simulink model "soc_dvbs2_fpga"  (R2025b)
settings: Solver=FixedStepDiscrete  StartTime=0.0  StopTime=0  RelTol=1e-3
InitFcn:
  | soc_dvbs2_init;
values from neighbouring files (symbols this model uses):
  Rsym = 4e6    (= 4000000)    [soc_dvbs2_init.m]
  soc_dvbs2_txPacketBits = [1 1 0 1 0 1 1 1 0 1 1 1 ... (2972 elements, 2972x1)]    [soc_dvbs2_txPacketBits.mat]
  syncWord = (dec2bin(hex2dec('AC')) - '0').'    [soc_dvbs2_init.m]
  txDataOut = txobj(frameBits(:))    [soc_dvbs2_init.m]
  txFiltCoeff = txobj.pTxFilterCoeff    [soc_dvbs2_init.m]
undefined symbols (not defined in the file or in its folder): Add, coefficientsLog, coefficientsSqrt1, coefficientsSqrt2, dataBits, designMultirateFIR, noisePow, NumBits1, NumBits2, seedsURNG1, seedsURNG2, Shift, Slope1, Slope2, soc_dvbs2_designFIRFilter, txDataOutS1, txDataOutS10, txDataOutS12, txDataOutS13, txDataOutS14, txDataOutS15, txDataOutS16, txDataOutS18, txDataOutS19, txDataOutS2, txDataOutS20, txDataOutS21, txDataOutS22, txDataOutS24, txDataOutS25, txDataOutS26, txDataOutS27, txDataOutS3, txDataOutS4, txDataOutS5, txDataOutS6, txDataOutS7, txDataOutS8, txDataOutS9
libraries: simulink x214, hdlsllib x211, dspsigops x22, dsphdlfiltering2 x8, dsphdlsigops2 x5, commseqgen3 x5, dsphdlmathfun2 x3, hwlogicconnlib x2, whdledac x2, commhdlcrc x2, whdlutilities x1, whdlmod x1
(part 2 of 12)

== system soc_dvbs2_fpga/DVBS2/DVBS2 TxRx/DVB-S2 HDL Receiver/No HDL2 ==
  UPL : Inport
  DFL : Inport  Port=2
  SYNC : Inport  Port=3
  SYNCD : Inport  Port=4
  frameStart : Inport  Port=5
  frameEnd : Inport  Port=6
  To Workspace : ToWorkspace  VariableName=simUPL  SampleTime=-1
      settings: Save2DSignal=2-D array (concatenate along first dimension)
  To Workspace1 : ToWorkspace  VariableName=simDFL  SampleTime=-1
      settings: Save2DSignal=2-D array (concatenate along first dimension)
  To Workspace2 : ToWorkspace  VariableName=simSYNC  SampleTime=-1
      settings: Save2DSignal=2-D array (concatenate along first dimension)
  To Workspace3 : ToWorkspace  VariableName=simSYNCD  SampleTime=-1
      settings: Save2DSignal=2-D array (concatenate along first dimension)
  To Workspace4 : ToWorkspace  VariableName=simFrameStart  SampleTime=-1
      settings: Save2DSignal=2-D array (concatenate along first dimension)
  To Workspace5 : ToWorkspace  VariableName=simFrameEnd  SampleTime=-1
      settings: Save2DSignal=2-D array (concatenate along first dimension)
  wires:
  DFL/1 -> To Workspace1/1
  SYNCD/1 -> To Workspace3/1
  UPL/1 -> To Workspace/1
  SYNC/1 -> To Workspace2/1
  frameStart/1 -> To Workspace4/1
  frameEnd/1 -> To Workspace5/1

== system soc_dvbs2_fpga/DVBS2/DVBS2 TxRx/DVB-S2 HDL Receiver/Stream Recovery ==
  bitsIn : Inport  OutDataTypeStr=boolean  PortDimensions=[1 1]  SampleTime=1/(Rsym*32)
  startIn : Inport  Port=2  OutDataTypeStr=boolean  PortDimensions=[1 1]
  validIn : Inport  Port=3  OutDataTypeStr=boolean  PortDimensions=[1 1]
  BB Decoder : Subsystem
      settings: PortSchema="{\"entries\":[{\"content\":{\"sides\":[{\"content\":{\"connectorIds\":[\"In1\",\"In2\",\"In3\",\"In4\",\"In5\",\"In6\",\"In7\",\"In8\"]},\"type\":\"ConnectorPlacement.EquallySpacedRectSide\",\"uuid\":\"2ee8952a-ba35-4074-ae69-b380b0fca75a\"},{\"content\":{\"connectorIds\":[\"Out1\",\"Out2\",\"Out3\",\"Out4\",\"Out5\",\"Out6\",\"Out7\",\"Out8\",\"Out9\",\"Out10\",\"Out11\",\"Out12\",\"Out13\",\"Out14\",\"Out15\",\"Out16\",\"Out17\"],\"side\":\"RIGHT\"},\"type\":\"ConnectorPlacement.EquallySpacedRectSide\",\"uuid\":\"5cd54040-f4d2-41eb-8bc9-10e507694db5\"},{\"content\":{\"connectorIds\":[\"Out18\",\"Out19\",\"Out20\"],\"side\":\"TOP\"},\"type\":\"ConnectorPlacement.EquallySpacedRectSide\",\"uuid\":\"7ef39af9-18b6-4154-ba4c-25b08baa09fa\"}]},\"type\":\"ConnectorPlacement.EquallySpacedConnector\",\"uuid\":\"52807250-24d4-4e44-a1d7-a664e63f1684\"}],\"packageUris\":[\"http://schema.mathworks.com/mf0/Connector/R2020b\"],\"version\":\"1.0\"}"
  BB Demultiplexer : Subsystem
  BB Descrambler : Subsystem
  BB Header CRC Check : Subsystem
  Delay{1..2,4..9,11..15,17..18,20..24} (20 alike) : Delay  DelayLength=1
  bitsOut : Outport  OutDataTypeStr=boolean  PortDimensions=[1 1]
  startOut : Outport  Port=2  OutDataTypeStr=boolean  PortDimensions=[1 1]
  endOut : Outport  Port=3  OutDataTypeStr=boolean  PortDimensions=[1 1]
  validOut : Outport  Port=4  OutDataTypeStr=boolean  PortDimensions=[1 1]
  errorOut : Outport  Port=5  OutDataTypeStr=boolean  PortDimensions=[1 1]
  invalidPkt : Outport  Port=6  OutDataTypeStr=boolean  PortDimensions=[1 1]
  headerCRCInfo : Outport  Port=7  OutDataTypeStr=fixdt(0,2,0)  PortDimensions=[1 1]
  TSorGS : Outport  Port=8  OutDataTypeStr=fixdt(0,2,0)  PortDimensions=[1 1]
  SISorMIS : Outport  Port=9  OutDataTypeStr=boolean  PortDimensions=[1 1]
  CCMorACM : Outport  Port=10  OutDataTypeStr=boolean  PortDimensions=[1 1]
  ISSYI : Outport  Port=11  OutDataTypeStr=boolean  PortDimensions=[1 1]
  NPD : Outport  Port=12  OutDataTypeStr=boolean  PortDimensions=[1 1]
  RO : Outport  Port=13  OutDataTypeStr=fixdt(0,2,0)  PortDimensions=[1 1]
  MIS_ISI : Outport  Port=14  OutDataTypeStr=uint8  PortDimensions=1
  UPL : Outport  Port=15  OutDataTypeStr=uint16  PortDimensions=1
  DFL : Outport  Port=16  OutDataTypeStr=uint16  PortDimensions=1
  SYNC : Outport  Port=17  OutDataTypeStr=uint8  PortDimensions=1
  SYNCD : Outport  Port=18  OutDataTypeStr=uint16  PortDimensions=1
  frameSrt : Outport  Port=19  OutDataTypeStr=boolean  PortDimensions=[1 1]
  frameEnd : Outport  Port=20  OutDataTypeStr=boolean  PortDimensions=[1 1]
  wires:
  bitsIn/1 -> Delay1/1
  BB Demultiplexer/2(dValidOut) -> Delay20/1
  BB Demultiplexer/6(hvalidOut) -> Delay24/1
  BB Decoder/5(errorOut) -> errorOut/1
  BB Decoder/4(validOut) -> validOut/1
  BB Decoder/1(bitsOut) -> bitsOut/1
  Delay9/1 -> BB Decoder/1(dstartIn)
  BB Descrambler/1(bitsOut) -> Delay7/1
  Delay14/1 -> BB Decoder/8(herrorIn)
  BB Decoder/8(SISorMIS) -> SISorMIS/1
  BB Header CRC Check/3(dbitsOut) -> Delay8/1
  Delay11/1 -> BB Decoder/2(dvalidIn)
  Delay8/1 -> BB Decoder/3(dbitsIn)
  BB Decoder/15(DFL) -> DFL/1
  BB Header CRC Check/8(herrorOut) -> Delay14/1
  Delay12/1 -> BB Decoder/7(validIn)
  BB Decoder/17(SYNCD) -> SYNCD/1
  BB Header CRC Check/4(hbitsOut) -> Delay13/1
  BB Decoder/11(NPD) -> NPD/1
  BB Demultiplexer/4(hstartOut) -> Delay22/1
  BB Decoder/12(RO) -> RO/1
  BB Demultiplexer/5(hendOut) -> Delay23/1
  BB Demultiplexer/1(dstartOut) -> Delay18/1
  BB Descrambler/3(validOut) -> Delay17/1
  validIn/1 -> Delay6/1
  BB Header CRC Check/7(hvalidOut) -> Delay12/1
  BB Decoder/14(UPL) -> UPL/1
  BB Decoder/3(endOut) -> endOut/1
  BB Decoder/9(CCMorACM) -> CCMorACM/1
  Delay4/1 -> BB Decoder/5(hstartIn)
  BB Demultiplexer/3(bitsOut) -> Delay21/1
  BB Descrambler/2(startOut) -> Delay15/1
  BB Header CRC Check/5(hstartOut) -> Delay4/1
  BB Header CRC Check/1(dstartOut) -> Delay9/1
  BB Decoder/2(startOut) -> startOut/1
  BB Decoder/10(ISSYI) -> ISSYI/1
  BB Header CRC Check/2(dvalidIn) -> Delay11/1
  BB Header CRC Check/6(hendOut) -> Delay5/1
  Delay5/1 -> BB Decoder/6(hendIn)
  Delay13/1 -> BB Decoder/4(hbitsIn)
  BB Decoder/13(MIS_ISI) -> MIS_ISI/1
  BB Decoder/16(SYNC) -> SYNC/1
  BB Decoder/7(TSorGS) -> TSorGS/1
  startIn/1 -> Delay2/1
  BB Decoder/18(invalidPkt) -> invalidPkt/1
  BB Decoder/6(headerCRCInfo) -> headerCRCInfo/1
  Delay1/1 -> BB Descrambler/1(bitsIn)
  Delay2/1 -> BB Descrambler/2(startIn)
  Delay6/1 -> BB Descrambler/3(validIn)
  Delay7/1 -> BB Demultiplexer/1(bitsIn)
  Delay15/1 -> BB Demultiplexer/2(startIn)
  Delay17/1 -> BB Demultiplexer/3(validIn)
  Delay18/1 -> BB Header CRC Check/1(dstartIn)
  Delay20/1 -> BB Header CRC Check/2(dValidIn)
  Delay21/1 -> BB Header CRC Check/3(bitsIn)
  Delay22/1 -> BB Header CRC Check/4(hstartIn)
  Delay23/1 -> BB Header CRC Check/5(hendIn)
  Delay24/1 -> BB Header CRC Check/6(hvalidIn)
  BB Decoder/19(frameStart) -> frameSrt/1
  BB Decoder/20(frameEnd) -> frameEnd/1

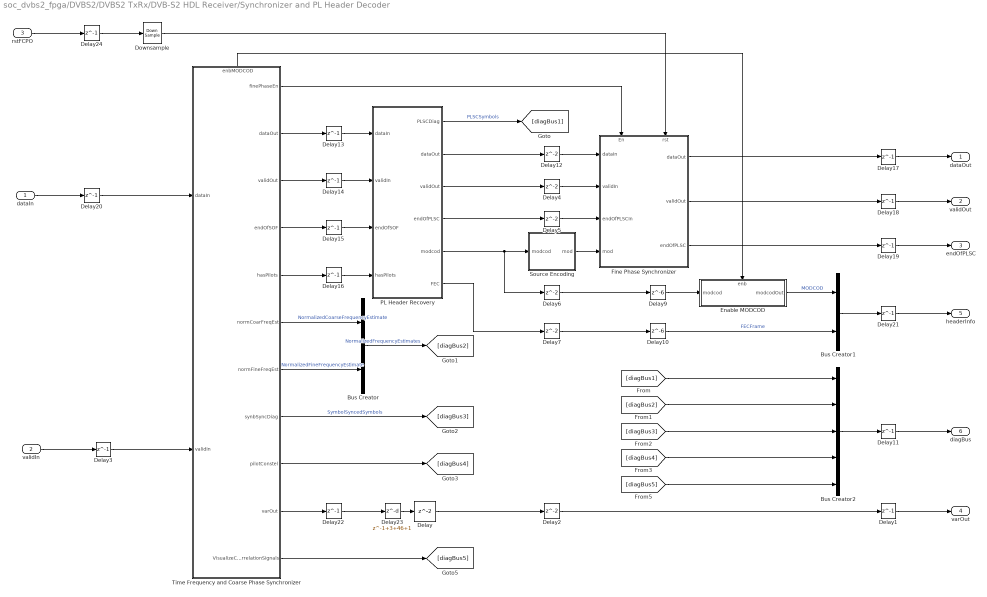
== system soc_dvbs2_fpga/DVBS2/DVBS2 TxRx/DVB-S2 HDL Receiver/Synchronizer and PL Header Decoder ==
  dataIn : Inport  OutDataTypeStr=fixdt(1,18,15)  PortDimensions=1  SampleTime=1/(Rsym*config.SamplesPerSymbol)
      settings: SignalType=complex
  validIn : Inport  Port=2  OutDataTypeStr=boolean  PortDimensions=1  SampleTime=1/(Rsym*config.SamplesPerSymbol)
  rstFCPO : Inport  Port=3  OutDataTypeStr=boolean  PortDimensions=1  SampleTime=1/(Rsym*config.SamplesPerSymbol)
  Bus Creator : BusCreator  Inputs=2
  Bus Creator1 : BusCreator  Inputs=2
  Bus Creator2 : BusCreator  Inputs=5
  Delay{,2,4..7,12} (7 alike) : Delay
  Delay{1,3,11,13..22,24} (14 alike) : Delay  DelayLength=1
  Delay10 : Delay  DelayLength=6
  Delay23 : Delay  DelayLength=1+3+46+1
  Delay9 : Delay  DelayLength=6
  Downsample : DownSample  N=config.SamplesPerSymbol  RateOptions=Allow multirate processing
  "Enable MODCOD " : Subsystem
      settings: PortSchema="{\"entries\":[{\"content\":{\"sides\":[{\"content\":{\"connectorIds\":[\"In1\"]},\"type\":\"ConnectorPlacement.EquallySpacedRectSide\",\"uuid\":\"e9d17376-cdb6-46fb-903f-9d282ad3c090\"},{\"content\":{\"connectorIds\":[\"Out1\"],\"side\":\"RIGHT\"},\"type\":\"ConnectorPlacement.EquallySpacedRectSide\",\"uuid\":\"a9734af5-b25e-45ab-96a0-7f27ff03e87c\"},{\"content\":{\"connectorIds\":[\"In2\"],\"side\":\"TOP\"},\"type\":\"ConnectorPlacement.EquallySpacedRectSide\",\"uuid\":\"cd34d4a9-2b51-417d-abe3-d9c0cedbfd72\"}]},\"type\":\"ConnectorPlacement.EquallySpacedConnector\",\"uuid\":\"3d42caf6-d237-4a2e-ba65-28be4744776a\"}],\"packageUris\":[\"http://schema.mathworks.com/mf0/Connector/R2020b\"],\"version\":\"1.0\"}"
      settings: LibrarySourceBlock=|
      | hdlsllib/Ports &
      | Subsystems/Subsystem
  Fine Phase Synchronizer : Subsystem
      settings: PortSchema="{\"entries\":[{\"content\":{\"sides\":[{\"content\":{\"connectorIds\":[\"In1\",\"In2\",\"In3\",\"In4\"]},\"type\":\"ConnectorPlacement.EquallySpacedRectSide\",\"uuid\":\"8cb05f70-3f7c-4fa6-8c33-963515007e67\"},{\"content\":{\"connectorIds\":[\"Out1\",\"Out2\",\"Out3\"],\"side\":\"RIGHT\"},\"type\":\"ConnectorPlacement.EquallySpacedRectSide\",\"uuid\":\"1928a8bf-9583-43f2-af59-80ea1a918df6\"},{\"content\":{\"connectorIds\":[\"In5\",\"In6\"],\"side\":\"TOP\"},\"type\":\"ConnectorPlacement.EquallySpacedRectSide\",\"uuid\":\"66048bc0-484a-4616-b173-7a52a6834176\"}]},\"type\":\"ConnectorPlacement.EquallySpacedConnector\",\"uuid\":\"51bb5bc9-87eb-4b94-8278-b6601d5ad231\"}],\"packageUris\":[\"http://schema.mathworks.com/mf0/Connector/R2020b\"],\"version\":\"1.0\"}"
  PL Header Recovery : Subsystem
  Source Encoding : Subsystem
  Time Frequency and Coarse Phase Synchronizer : Subsystem
      settings: PortSchema="{\"entries\":[{\"content\":{\"sides\":[{\"content\":{\"connectorIds\":[\"In1\",\"In2\"]},\"type\":\"ConnectorPlacement.EquallySpacedRectSide\",\"uuid\":\"4d277405-2c1f-464d-b6dc-b1e9ab229e6e\"},{\"content\":{\"connectorIds\":[\"Out1\",\"Out2\",\"Out3\",\"Out4\",\"Out5\",\"Out6\",\"Out7\",\"Out8\",\"Out9\",\"Out10\",\"Out11\"],\"side\":\"RIGHT\"},\"type\":\"ConnectorPlacement.EquallySpacedRectSide\",\"uuid\":\"271739cd-2ba1-4a70-9167-bfb95088c1ca\"},{\"content\":{\"connectorIds\":[\"Out12\"],\"side\":\"TOP\"},\"type\":\"ConnectorPlacement.EquallySpacedRectSide\",\"uuid\":\"6ccba931-85ed-495e-b91c-84f6ac00e636\"}]},\"type\":\"ConnectorPlacement.EquallySpacedConnector\",\"uuid\":\"210794f0-4960-4096-827d-5c263124cba0\"}],\"packageUris\":[\"http://schema.mathworks.com/mf0/Connector/R2020b\"],\"version\":\"1.0\"}"
  dataOut : Outport
  validOut : Outport  Port=2
  endOfPLSC : Outport  Port=3
  varOut : Outport  Port=4
  headerInfo : Outport  Port=5
  diagBus : Outport  Port=6
  wires:
  Bus Creator2/1 -> Delay11/1
  [diagBus4] -> Bus Creator2/4
  PL Header Recovery/6(FEC) -> Delay7/1
  Time Frequency and Coarse Phase Synchronizer/5(hasPilots) -> Delay16/1
  Time Frequency and Coarse Phase Synchronizer/10(varOut) -> Delay22/1
  Bus Creator1/1 -> Delay21/1
  Delay9/1 -> "Enable MODCOD "/1(modcod)
  rstFCPO/1 -> Delay24/1
  PL Header Recovery/5(modcod) -> Source Encoding/1(modcod), Delay6/1
  Delay13/1 -> PL Header Recovery/1(dataIn)
  [diagBus1] -> Bus Creator2/1
  Delay22/1 -> Delay23/1
  Delay19/1 -> endOfPLSC/1
  PL Header Recovery/3(validOut) -> Delay4/1
  [diagBus5] -> Bus Creator2/5
  Delay12/1 -> Fine Phase Synchronizer/1(dataIn)
  Delay10/1 -> Bus Creator1/2  "FECFrame"
  Fine Phase Synchronizer/1(dataOut) -> Delay17/1
  validIn/1 -> Delay3/1
  Fine Phase Synchronizer/3(endOfPLSC) -> Delay19/1
  PL Header Recovery/2(dataOut) -> Delay12/1
  Time Frequency and Coarse Phase Synchronizer/2(dataOut) -> Delay13/1
  dataIn/1 -> Delay20/1
  Time Frequency and Coarse Phase Synchronizer/11(VisualizeCorrelationSignals) -> [diagBus5]
  Delay7/1 -> Delay10/1
  Delay14/1 -> PL Header Recovery/2(validIn)
  Time Frequency and Coarse Phase Synchronizer/4(endOfSOF) -> Delay15/1
  Fine Phase Synchronizer/2(validOut) -> Delay18/1
  Delay5/1 -> Fine Phase Synchronizer/3(endOfPLSCIn)
  Delay3/1 -> Time Frequency and Coarse Phase Synchronizer/2(validIn)
  Delay/1 -> Delay2/1
  Time Frequency and Coarse Phase Synchronizer/3(validOut) -> Delay14/1
  Delay16/1 -> PL Header Recovery/4(hasPilots)
  [diagBus2] -> Bus Creator2/2
  Delay2/1 -> Delay1/1
  Delay15/1 -> PL Header Recovery/3(endOfSOF)
  Delay6/1 -> Delay9/1
  Delay17/1 -> dataOut/1
  PL Header Recovery/4(endOfPLSC) -> Delay5/1
  [diagBus3] -> Bus Creator2/3
  Delay4/1 -> Fine Phase Synchronizer/2(validIn)
  Source Encoding/1(mod) -> Fine Phase Synchronizer/4(mod)
  Delay18/1 -> validOut/1
  Time Frequency and Coarse Phase Synchronizer/8(synbSyncDiag) -> [diagBus3]  "SymbolSyncedSymbols"
  PL Header Recovery/1(PLSCDiag) -> [diagBus1]  "PLSCSymbols"
  Time Frequency and Coarse Phase Synchronizer/1(finePhaseEn) -> Fine Phase Synchronizer/5(En)
  Time Frequency and Coarse Phase Synchronizer/9(pilotConstel) -> [diagBus4]
  Delay1/1 -> varOut/1
  Delay20/1 -> Time Frequency and Coarse Phase Synchronizer/1(dataIn)
  Delay23/1 -> Delay/1
  Delay24/1 -> Downsample/1
  Delay11/1 -> diagBus/1
  Delay21/1 -> headerInfo/1
  Downsample/1 -> Fine Phase Synchronizer/6(rst)
  "Enable MODCOD "/1(modcodOut) -> Bus Creator1/1  "MODCOD"
  Time Frequency and Coarse Phase Synchronizer/12(enbMODCOD) -> "Enable MODCOD "/2(enb)
  Bus Creator/1 -> [diagBus2]  "NormalizedFrequencyEstimates"
  Time Frequency and Coarse Phase Synchronizer/6(normCoarFreqEst) -> Bus Creator/1  "NormalizedCoarseFrequencyEstimate"
  Time Frequency and Coarse Phase Synchronizer/7(normFineFreqEst) -> Bus Creator/2  "NormalizedFineFrequencyEstimate"

== system soc_dvbs2_fpga/DVBS2/DVBS2 TxRx/Digital Automatic Gain Control/Error Detector ==
  dataIn : Inport
  Add1 : Sum  Inputs=+-
  Complex to Real-Imag : ComplexToRealImag  Output=Real
  Conj : Math  Operator=conj
  Data Type Duplicate : DataTypeDuplicate
  Delay{,1,3..4} (4 alike) : Delay
  Product : Product
  Reference : Constant  Value=desiredOutputPower  OutDataTypeStr=Inherit: Inherit via back propagation  SampleTime=-1
  err : Outport
  wires:
  Complex to Real-Imag/1 -> Add1/2
  Product/1 -> Delay4/1
  Delay4/1 -> Complex to Real-Imag/1
  Delay3/1 -> err/1
  Delay1/1 -> Product/1
  Delay/1 -> Product/2
  Reference/1 -> Add1/1, Data Type Duplicate/1
  Conj/1 -> Delay/1
  dataIn/1 -> Conj/1, Data Type Duplicate/2, Delay1/1
  Add1/1 -> Delay3/1

== system soc_dvbs2_fpga/DVBS2/DVBS2 TxRx/Digital Automatic Gain Control/Loop Filter ==
  note: Fixed point precision loss warnings
      | are supressed in Mask Init Callback
  err : Inport
  Add : Sum  Inputs=|++  OutDataTypeStr=Inherit: Same as first input
  Delay1 : Delay  DelayLength=1
  Delay2 : Delay
  Delay3 : Delay
  Gain1 : Gain  Gain=stepSize  OutDataTypeStr=Inherit: Same as input
      mask init:
      | Simulink.suppressDiagnostic(gcb, 'SimulinkFixedPoint:util:fxpParameterPrecisionLoss');
  gain : Outport
  wires:
  Delay3/1 -> Gain1/1
  Delay2/1 -> Add/1
  Gain1/1 -> Delay2/1
  Add/1 -> Delay1/1
  Delay1/1 -> Add/2, gain/1
  err/1 -> Delay3/1

== system soc_dvbs2_fpga/DVBS2/DVBS2 TxRx/LUT Based Tx/Subsystem1 ==
  modcodidx : Inport
  enb : Inport  Port=2
  Delay : Delay  DelayLength=1
  From : From
  Goto : Goto
  HDL Counter : hdlsllib/Sources/HDL Counter  CountType=Count limited  CountInit=0  CountStep=1  CountMax=8370-1  CountFromType=Initial value  CountFrom=0  CountResetPort=off  CountLoadPort=off  CountEnbPort=on  CountDirPort=off  CountHitOutputPort=off  CountDataType=Unsigned  CountWordLen=32  CountFracLen=0  CountSampTime=1
  Logical Operator : Logic  Operator=OR  Inputs=4  AllPortsSameDT=off  OutDataTypeStr=boolean
  Multiport Switch : MultiPortSwitch  DataPortOrder=Zero-based contiguous  Inputs=24  DataPortForDefault=Additional data port  DiagnosticForDefault=Warning  zeroidx=on  SaturateOnIntegerOverflow=off  InputSameDT=off
  Subsystem : Subsystem
      settings: PortSchema="{\"entries\":[{\"content\":{\"sides\":[{\"content\":{\"connectorIds\":[\"In1\",\"In2\",\"In3\"]},\"type\":\"ConnectorPlacement.EquallySpacedRectSide\",\"uuid\":\"6ed0080d-8044-45ae-9509-1be5017662ca\"},{\"content\":{\"connectorIds\":[\"Out1\",\"Out2\",\"Out3\",\"Out4\",\"Out5\",\"Out6\"],\"side\":\"RIGHT\"},\"type\":\"ConnectorPlacement.EquallySpacedRectSide\",\"uuid\":\"674d766f-0d57-4001-a79f-bea5e47ca454\"},{\"content\":{\"connectorIds\":[\"Out7\"],\"side\":\"TOP\"},\"type\":\"ConnectorPlacement.EquallySpacedRectSide\",\"uuid\":\"4af606e0-b38a-47a9-8ca6-549744415caf\"}]},\"type\":\"ConnectorPlacement.EquallySpacedConnector\",\"uuid\":\"5c295423-4673-440c-afff-1364a30dca72\"}],\"packageUris\":[\"http://schema.mathworks.com/mf0/Connector/R2020b\"],\"version\":\"1.0\"}"
  Subsystem1 : Subsystem
      settings: PortSchema="{\"entries\":[{\"content\":{\"sides\":[{\"content\":{\"connectorIds\":[\"In1\",\"In2\",\"In3\"]},\"type\":\"ConnectorPlacement.EquallySpacedRectSide\",\"uuid\":\"6ed0080d-8044-45ae-9509-1be5017662ca\"},{\"content\":{\"connectorIds\":[\"Out1\",\"Out2\",\"Out3\",\"Out4\",\"Out5\",\"Out6\"],\"side\":\"RIGHT\"},\"type\":\"ConnectorPlacement.EquallySpacedRectSide\",\"uuid\":\"674d766f-0d57-4001-a79f-bea5e47ca454\"},{\"content\":{\"connectorIds\":[\"Out7\"],\"side\":\"TOP\"},\"type\":\"ConnectorPlacement.EquallySpacedRectSide\",\"uuid\":\"4af606e0-b38a-47a9-8ca6-549744415caf\"}]},\"type\":\"ConnectorPlacement.EquallySpacedConnector\",\"uuid\":\"5c295423-4673-440c-afff-1364a30dca72\"}],\"packageUris\":[\"http://schema.mathworks.com/mf0/Connector/R2020b\"],\"version\":\"1.0\"}"
  Subsystem2 : Subsystem
      settings: PortSchema="{\"entries\":[{\"content\":{\"sides\":[{\"content\":{\"connectorIds\":[\"In1\",\"In2\",\"In3\"]},\"type\":\"ConnectorPlacement.EquallySpacedRectSide\",\"uuid\":\"6ed0080d-8044-45ae-9509-1be5017662ca\"},{\"content\":{\"connectorIds\":[\"Out1\",\"Out2\",\"Out3\",\"Out4\",\"Out5\",\"Out6\"],\"side\":\"RIGHT\"},\"type\":\"ConnectorPlacement.EquallySpacedRectSide\",\"uuid\":\"674d766f-0d57-4001-a79f-bea5e47ca454\"},{\"content\":{\"connectorIds\":[\"Out7\"],\"side\":\"TOP\"},\"type\":\"ConnectorPlacement.EquallySpacedRectSide\",\"uuid\":\"4af606e0-b38a-47a9-8ca6-549744415caf\"}]},\"type\":\"ConnectorPlacement.EquallySpacedConnector\",\"uuid\":\"5c295423-4673-440c-afff-1364a30dca72\"}],\"packageUris\":[\"http://schema.mathworks.com/mf0/Connector/R2020b\"],\"version\":\"1.0\"}"
  Subsystem4 : Subsystem
      settings: PortSchema="{\"entries\":[{\"content\":{\"sides\":[{\"content\":{\"connectorIds\":[\"In1\",\"In2\",\"In3\"]},\"type\":\"ConnectorPlacement.EquallySpacedRectSide\",\"uuid\":\"6ed0080d-8044-45ae-9509-1be5017662ca\"},{\"content\":{\"connectorIds\":[\"Out1\",\"Out2\",\"Out3\",\"Out4\",\"Out5\",\"Out6\"],\"side\":\"RIGHT\"},\"type\":\"ConnectorPlacement.EquallySpacedRectSide\",\"uuid\":\"674d766f-0d57-4001-a79f-bea5e47ca454\"},{\"content\":{\"connectorIds\":[\"Out7\"],\"side\":\"TOP\"},\"type\":\"ConnectorPlacement.EquallySpacedRectSide\",\"uuid\":\"4af606e0-b38a-47a9-8ca6-549744415caf\"}]},\"type\":\"ConnectorPlacement.EquallySpacedConnector\",\"uuid\":\"5c295423-4673-440c-afff-1364a30dca72\"}],\"packageUris\":[\"http://schema.mathworks.com/mf0/Connector/R2020b\"],\"version\":\"1.0\"}"
  Terminator : Terminator
  Unit Delay Enabled Synchronous : hdlsllib/Discrete/Unit Delay Enabled Synchronous  InitialCondition=0.0  SampleTime=-1
  Out1 : Outport
  wires:
  Unit Delay Enabled Synchronous/1 -> Goto/1, Multiport Switch/1
  Multiport Switch/1 -> Out1/1
  modcodidx/1 -> Unit Delay Enabled Synchronous/1
  Delay/1 -> Subsystem2/1(rst), Subsystem4/1(rst), Subsystem1/1(rst), Subsystem/1(rst)
  enb/1 -> HDL Counter/1, Subsystem/2(enb), Subsystem2/2(enb), Subsystem4/2(enb), Subsystem1/2(enb)
  Subsystem/1(Out2) -> Multiport Switch/2, Multiport Switch/26
  Subsystem/2(Out3) -> Multiport Switch/3
  Subsystem/3(Out4) -> Multiport Switch/4
  Subsystem/4(Out5) -> Multiport Switch/5
  Subsystem/5(Out6) -> Multiport Switch/6
  Subsystem/6(Out7) -> Multiport Switch/7
  Subsystem1/1(Out2) -> Multiport Switch/8
  Subsystem1/2(Out3) -> Multiport Switch/9
  Subsystem1/3(Out4) -> Multiport Switch/10
  Subsystem1/4(Out5) -> Multiport Switch/11
  Subsystem1/5(Out6) -> Multiport Switch/12
  Subsystem1/6(Out7) -> Multiport Switch/13
  Subsystem4/1(Out2) -> Multiport Switch/14
  Subsystem4/2(Out3) -> Multiport Switch/15
  Subsystem4/3(Out4) -> Multiport Switch/16
  Subsystem4/4(Out5) -> Multiport Switch/17
  Subsystem4/5(Out6) -> Multiport Switch/18
  Subsystem4/6(Out7) -> Multiport Switch/19
  Subsystem2/1(Out2) -> Multiport Switch/20
  Subsystem2/2(Out3) -> Multiport Switch/21
  Subsystem2/3(Out4) -> Multiport Switch/22
  Subsystem2/4(Out5) -> Multiport Switch/23
  Subsystem2/5(Out6) -> Multiport Switch/24
  Subsystem2/6(Out7) -> Multiport Switch/25
  Logical Operator/1 -> Unit Delay Enabled Synchronous/2, Delay/1
  Subsystem/7(Out1) -> Logical Operator/1
  Subsystem4/7(Out1) -> Logical Operator/2
  Subsystem1/7(Out1) -> Logical Operator/3
  Subsystem2/7(Out1) -> Logical Operator/4
  From/1 -> Subsystem2/3(modcodidx), Subsystem4/3(modcodidx), Subsystem1/3(modcodidx), Subsystem/3(modcodidx)
  HDL Counter/1 -> Terminator/1

== system soc_dvbs2_fpga/DVBS2/DVBS2 TxRx/Channel/AWGN Generator/Gaussian Noise With Given Variance ==
  noiseVar : Inport
  x0 : Inport  Port=2
  x1 : Inport  Port=3
  Add1 : Sum  OutDataTypeStr=fixdt(1,16,11)
  Delay{1..9} (9 alike) : Delay
  Gain : Gain  Gain=1i
  Product1 : Product
  awgn : Outport
  wires:
  Add1/1 -> Delay3/1
  Product1/1 -> Delay1/1
  x1/1 -> Delay9/1
  x0/1 -> Delay8/1
  Gain/1 -> Delay5/1
  noiseVar/1 -> Delay7/1
  Delay1/1 -> awgn/1
  Delay2/1 -> Product1/1
  Delay3/1 -> Product1/2
  Delay4/1 -> Add1/1
  Delay5/1 -> Add1/2
  Delay6/1 -> Delay2/1
  Delay7/1 -> Delay6/1
  Delay8/1 -> Delay4/1
  Delay9/1 -> Gain/1

== system soc_dvbs2_fpga/DVBS2/DVBS2 TxRx/Channel/AWGN Generator/Unit Variance Gaussian Noise ==
  Delay{,1..2,31,33} (5 alike) : Delay  DelayLength=1
  Delay{5..10} (6 alike) : Delay
  Delay23 : Delay  DelayLength=19
  Delay24 : Delay  DelayLength=19
  Delay3 : Delay  DelayLength=21
  Delay4 : Delay  DelayLength=21
  Product : Product  OutDataTypeStr=fixdt(1,16,11)
  Product1 : Product  OutDataTypeStr=fixdt(1,16,11)
  SinCos : Subsystem
  SqrtImplementation : Subsystem
  TausUniformRandGen : Subsystem
  logImplementation : Subsystem
  x0 : Outport
  x1 : Outport  Port=2
  wires:
  TausUniformRandGen/2(u1(16,16)) -> Delay2/1
  logImplementation/1(e) -> Delay1/1
  Product/1 -> Delay9/1  "x0(16,11)"
  Product1/1 -> Delay10/1  "x1(16,11)"
  Delay24/1 -> Delay8/1
  Delay23/1 -> Delay6/1
  Delay31/1 -> Delay23/1
  Delay33/1 -> Delay24/1
  SqrtImplementation/1(f) -> Delay5/1, Delay7/1
  TausUniformRandGen/1(u0(16,16)) -> Delay/1
  SinCos/1(g0) -> Delay3/1
  SinCos/2(g1(16,15)) -> Delay4/1
  Delay1/1 -> SqrtImplementation/1(u)
  Delay/1 -> logImplementation/1(u0(48,48))
  Delay2/1 -> SinCos/1(u1)
  Delay3/1 -> Delay31/1
  Delay4/1 -> Delay33/1
  Delay5/1 -> Product/1
  Delay6/1 -> Product/2
  Delay7/1 -> Product1/1
  Delay8/1 -> Product1/2
  Delay9/1 -> x0/1
  Delay10/1 -> x1/1

== system soc_dvbs2_fpga/DVBS2/DVBS2 TxRx/Channel/AWGN Generator/dB to Linear Scale Converter ==
  note: Add Block is used to obtain integer index to Lookup Table
  snrdB : Inport
  Add : Sum  OutDataTypeStr=int16
  Constant : Constant  Value=201  OutDataTypeStr=int16  SampleTime=-1
  Delay{1..4} (4 alike) : Delay
  Delay5 : Delay  DelayLength=1
  Delay6 : Delay  DelayLength=1
  Gain : Gain  Gain=10  OutDataTypeStr=int16  RndMeth=Round
  sqrt(noisePow/2) : Lookup_n-D  NumberOfTableDimensions=1  LookupTableObject=''  BreakpointsForDimension1=0:511  BreakpointsForDimension1FirstPoint=10  BreakpointsForDimension2FirstPoint=10  BreakpointsForDimension1Spacing=12  BreakpointsForDimension2Spacing=12  IndexSearchMethod=Evenly spaced points  Table=[0 noisePow]  InterpMethod=Flat  DiagnosticForOutOfRangeInput=Error  InternalRulePriority=Speed  OutDataTypeStr=fixdt(0,22,18)  RndMeth=Simplest
  noiseVar : Outport
  wires:
  Gain/1 -> Delay3/1
  sqrt(noisePow/2)/1 -> Delay4/1
  Constant/1 -> Add/2
  Delay1/1 -> sqrt(noisePow/2)/1
  snrdB/1 -> Delay5/1
  Delay2/1 -> Gain/1
  Delay3/1 -> Add/1
  Delay4/1 -> Delay6/1
  Add/1 -> Delay1/1
  Delay6/1 -> noiseVar/1
  Delay5/1 -> Delay2/1

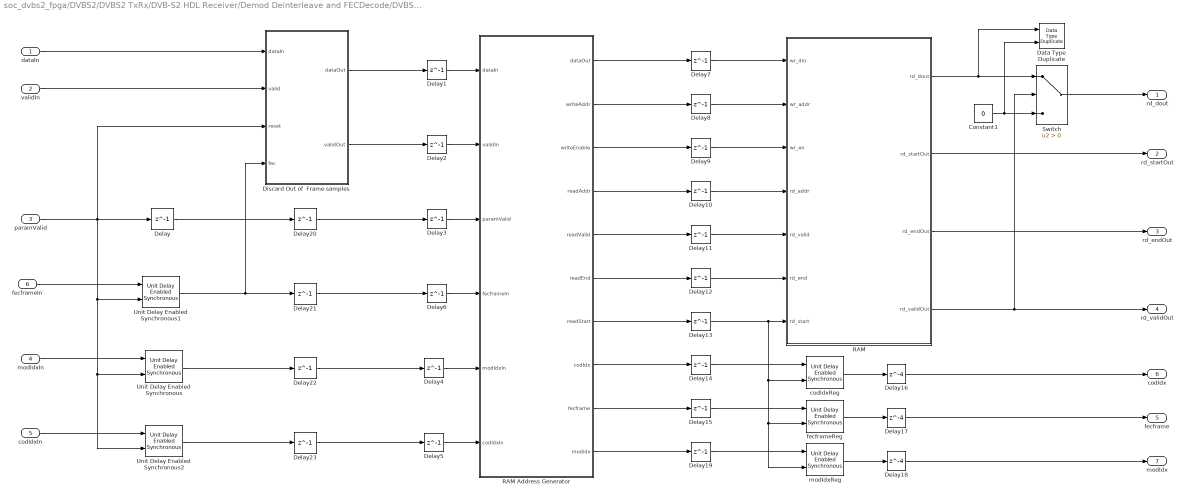
== system soc_dvbs2_fpga/DVBS2/DVBS2 TxRx/DVB-S2 HDL Receiver/Demod Deinterleave and FECDecode/DVBS2 HDL Deinterleaver ==
  dataIn : Inport
  validIn : Inport  Port=2
  paramValid : Inport  Port=3
  modIdxIn : Inport  Port=4
  codIdxIn : Inport  Port=5
  fecframeIn : Inport  Port=6
  Constant1 : Constant  Value=0  OutDataTypeStr=Inherit: Inherit via back propagation  SampleTime=Tsamp
  Data Type Duplicate : DataTypeDuplicate
  Delay{,1..15,19..23} (21 alike) : Delay  DelayLength=1
  Delay16 : Delay  DelayLength=4
  Delay17 : Delay  DelayLength=4
  Delay18 : Delay  DelayLength=4
  Discard Out of  Frame samples : MATLAB Function  TreatAsAtomicUnit=on
  RAM : Subsystem
  RAM Address Generator : Subsystem
  Switch : Switch  Criteria=u2 > Threshold  SaturateOnIntegerOverflow=off  InputSameDT=off
  Unit Delay Enabled Synchronous : hdlsllib/Discrete/Unit Delay Enabled Synchronous  InitialCondition=0.0  SampleTime=-1
  Unit Delay Enabled Synchronous1 : hdlsllib/Discrete/Unit Delay Enabled Synchronous  InitialCondition=0.0  SampleTime=-1
  Unit Delay Enabled Synchronous2 : hdlsllib/Discrete/Unit Delay Enabled Synchronous  InitialCondition=0.0  SampleTime=-1
  codIdxReg : hdlsllib/Discrete/Unit Delay Enabled Synchronous  InitialCondition=0.0  SampleTime=-1
  fecframeReg : hdlsllib/Discrete/Unit Delay Enabled Synchronous  InitialCondition=0.0  SampleTime=-1
  modIdxReg : hdlsllib/Discrete/Unit Delay Enabled Synchronous  InitialCondition=0.0  SampleTime=-1
  rd_dout : Outport
  rd_startOut : Outport  Port=2
  rd_endOut : Outport  Port=3
  rd_validOut : Outport  Port=4
  fecframe : Outport  Port=5
  codIdx : Outport  Port=6
  modIdx : Outport  Port=7
  wires:
  Delay17/1 -> fecframe/1
  Delay16/1 -> codIdx/1
  Delay15/1 -> fecframeReg/1
  Delay14/1 -> codIdxReg/1
  Delay13/1 -> codIdxReg/2, modIdxReg/2, fecframeReg/2, RAM/7(rd_start)
  Delay12/1 -> RAM/6(rd_end)
  Delay11/1 -> RAM/5(rd_valid)
  Delay10/1 -> RAM/4(rd_addr)
  Delay9/1 -> RAM/3(wr_en)
  Delay8/1 -> RAM/2(wr_addr)
  Delay7/1 -> RAM/1(wr_din)
  Delay6/1 -> RAM Address Generator/4(fecframeIn)
  Delay5/1 -> RAM Address Generator/6(codIdxIn)
  Delay4/1 -> RAM Address Generator/5(modIdxIn)
  Delay3/1 -> RAM Address Generator/3(paramValid)
  Delay2/1 -> RAM Address Generator/2(validIn)
  Delay1/1 -> RAM Address Generator/1(dataIn)
  codIdxReg/1 -> Delay16/1
  RAM/1(rd_dout) -> Data Type Duplicate/1, Switch/1
  fecframeReg/1 -> Delay17/1
  RAM/2(rd_startOut) -> rd_startOut/1
  RAM/3(rd_endOut) -> rd_endOut/1
  fecframeIn/1 -> Unit Delay Enabled Synchronous1/1
  modIdxIn/1 -> Unit Delay Enabled Synchronous/1
  codIdxIn/1 -> Unit Delay Enabled Synchronous2/1
  paramValid/1 -> Discard Out of  Frame samples/3(reset), Delay/1, Unit Delay Enabled Synchronous2/2, Unit Delay Enabled Synchronous/2, Unit Delay Enabled Synchronous1/2
  RAM/4(rd_validOut) -> Switch/2, rd_validOut/1
  validIn/1 -> Discard Out of  Frame samples/2(valid)
  RAM Address Generator/1(dataOut) -> Delay7/1
  dataIn/1 -> Discard Out of  Frame samples/1(dataIn)
  RAM Address Generator/3(writeEnable) -> Delay9/1
  RAM Address Generator/9(fecframe) -> Delay15/1
  RAM Address Generator/6(readEnd) -> Delay12/1
  RAM Address Generator/7(readStart) -> Delay13/1
  RAM Address Generator/4(readAddr) -> Delay10/1
  RAM Address Generator/2(writeAddr) -> Delay8/1
  RAM Address Generator/8(codIdx) -> Delay14/1
  RAM Address Generator/5(readValid) -> Delay11/1
  modIdxReg/1 -> Delay18/1
  Delay18/1 -> modIdx/1
  RAM Address Generator/10(modidx) -> Delay19/1
  Delay19/1 -> modIdxReg/1
  Delay/1 -> Delay20/1
  Unit Delay Enabled Synchronous1/1 -> Discard Out of  Frame samples/4(fec), Delay21/1
  Unit Delay Enabled Synchronous2/1 -> Delay23/1
  Unit Delay Enabled Synchronous/1 -> Delay22/1
  Discard Out of  Frame samples/2(validOut) -> Delay2/1
  Switch/1 -> rd_dout/1
  Constant1/1 -> Data Type Duplicate/2, Switch/3
  Discard Out of  Frame samples/1(dataOut) -> Delay1/1
  Delay20/1 -> Delay3/1
  Delay21/1 -> Delay6/1
  Delay22/1 -> Delay4/1
  Delay23/1 -> Delay5/1

== system soc_dvbs2_fpga/DVBS2/DVBS2 TxRx/DVB-S2 HDL Receiver/Demod Deinterleave and FECDecode/Discard Unsupported Frames ==
  endOfPLSC : Inport
  dataIn : Inport  Port=2
  validIn : Inport  Port=3
  nVarIn : Inport  Port=4
  MODCOD : Inport  Port=5
  FECFrame : Inport  Port=6
  Compare To Constant : simulink/Logic and Bit Operations/Compare To Constant  relop===  const=0  OutDataTypeStr=boolean
  Compare To Constant1 : simulink/Logic and Bit Operations/Compare To Constant  relop===  const=11  OutDataTypeStr=boolean
  Compare To Constant2 : simulink/Logic and Bit Operations/Compare To Constant  relop===  const=17  OutDataTypeStr=boolean
  Compare To Constant3 : simulink/Logic and Bit Operations/Compare To Constant  relop===  const=23  OutDataTypeStr=boolean
  Compare To Constant4 : simulink/Logic and Bit Operations/Compare To Constant  relop===  const=28  OutDataTypeStr=boolean
  Compare To Constant5 : simulink/Logic and Bit Operations/Compare To Constant  relop=>  const=28  OutDataTypeStr=boolean
  Constant : Constant  Value=complex(0)  OutDataTypeStr=Inherit: Inherit via back propagation  SampleTime=-1
  Constant1 : Constant  Value=FECFrameConst  OutDataTypeStr=boolean  SampleTime=-1
  Data Type Duplicate : DataTypeDuplicate
  Data Type Conversion : DataTypeConversion  OutDataTypeStr=fixdt(0,2,0)  SaturateOnIntegerOverflow=off  RndMeth=Floor
  Data Type Conversion1 : DataTypeConversion  OutDataTypeStr=fixdt(0,4,0)  SaturateOnIntegerOverflow=off  RndMeth=Floor
  Delay{,1..9} (10 alike) : Delay  DelayLength=1
  Delay10 : Delay  DelayLength=8
  Logical Operator : Logic  Operator=OR  Inputs=4  AllPortsSameDT=off  OutDataTypeStr=boolean
  Logical Operator1 : Logic  AllPortsSameDT=off  OutDataTypeStr=boolean
  Logical Operator2 : Logic  AllPortsSameDT=off  OutDataTypeStr=boolean
  Logical Operator3 : Logic  Operator=OR  AllPortsSameDT=off  OutDataTypeStr=boolean
  Logical Operator4 : Logic  Operator=OR  AllPortsSameDT=off  OutDataTypeStr=boolean
  Logical Operator5 : Logic  AllPortsSameDT=off  OutDataTypeStr=boolean
  Switch : Switch  Criteria=u2 ~= 0  SaturateOnIntegerOverflow=off  InputSameDT=off
  Terminator1 : Terminator
  Unit Delay Enabled Synchronous : hdlsllib/Discrete/Unit Delay Enabled Synchronous  InitialCondition=0.0  SampleTime=-1
  Unit Delay Enabled Synchronous1 : hdlsllib/Discrete/Unit Delay Enabled Synchronous  InitialCondition=0.0  SampleTime=-1
  Unit Delay Enabled Resettable Synchronous : hdlsllib/Discrete/Unit Delay Enabled Resettable Synchronous  InitialCondition=0.0  SampleTime=-1
  convertMODCOD : MATLAB Function  TreatAsAtomicUnit=on
  dataOut : Outport
  validOut : Outport  Port=2
  nVarOut : Outport  Port=3
  paramCapture : Outport  Port=4
  modIdx : Outport  Port=5
  codIdx : Outport  Port=6
  FECFrameOut : Outport  Port=7
  wires:
  Unit Delay Enabled Synchronous/1 -> Compare To Constant/1, Compare To Constant5/1, Compare To Constant1/1, Compare To Constant2/1, Compare To Constant3/1, Compare To Constant4/1, Delay3/1
  Delay6/1 -> Delay8/1
  Delay5/1 -> Delay4/1
  Delay8/1 -> Data Type Duplicate/1, Switch/1
  Delay2/1 -> FECFrameOut/1
  Unit Delay Enabled Synchronous1/1 -> Logical Operator1/2, Delay2/1
  convertMODCOD/1(modIdx) -> Data Type Conversion/1
  Delay7/1 -> Unit Delay Enabled Resettable Synchronous/2, Unit Delay Enabled Resettable Synchronous/1, Delay9/1
  Delay/1 -> Delay1/1
  nVarIn/1 -> Delay/1
  MODCOD/1 -> Unit Delay Enabled Synchronous/1
  validIn/1 -> Delay5/1
  dataIn/1 -> Delay6/1
  FECFrame/1 -> Terminator1/1
  endOfPLSC/1 -> Delay10/1
  Compare To Constant1/1 -> Logical Operator/1
  Compare To Constant2/1 -> Logical Operator/2
  Compare To Constant3/1 -> Logical Operator/3
  Compare To Constant4/1 -> Logical Operator/4
  Unit Delay Enabled Resettable Synchronous/1 -> Logical Operator5/2, Logical Operator2/2
  Logical Operator2/1 -> validOut/1, Switch/2
  Logical Operator/1 -> Logical Operator1/1
  Logical Operator1/1 -> Logical Operator3/2
  Compare To Constant/1 -> Logical Operator4/1
  Compare To Constant5/1 -> Logical Operator4/2
  Logical Operator4/1 -> Logical Operator3/1
  Logical Operator3/1 -> Unit Delay Enabled Resettable Synchronous/3
  Delay1/1 -> nVarOut/1
  Delay3/1 -> convertMODCOD/1(modcod)
  Delay4/1 -> Logical Operator2/1
  Delay9/1 -> Logical Operator5/1
  Switch/1 -> dataOut/1
  Constant/1 -> Data Type Duplicate/2, Switch/3
  Delay10/1 -> Unit Delay Enabled Synchronous/2, Unit Delay Enabled Synchronous1/2, Delay7/1
  convertMODCOD/2(codIdx) -> Data Type Conversion1/1
  Constant1/1 -> Unit Delay Enabled Synchronous1/1
  Logical Operator5/1 -> paramCapture/1
  Data Type Conversion/1 -> modIdx/1
  Data Type Conversion1/1 -> codIdx/1

== system soc_dvbs2_fpga/DVBS2/DVBS2 TxRx/DVB-S2 HDL Receiver/Demod Deinterleave and FECDecode/FEC Decoding ==
  dataIn : Inport
  startIn : Inport  Port=2
  endIn : Inport  Port=3
  validIn : Inport  Port=4
  FECFrame : Inport  Port=5
  codIdx : Inport  Port=6
  Bus Selector : BusSelector  OutputSignals=start
  DVB-S2 BCH Decoder : whdledac/DVB-S2 BCH Decoder  FECFrameSource=Property  FECFrameType=Short  CodeRateSource=Input port  CodeRateNormal=1/4  CodeRateShort=1/4  NumErrorsOutputPort=off  SimulateUsing=Code generation
  DVB-S2 LDPC Decoder : whdledac/DVB-S2 LDPC Decoder  FECFrameSource=Input port  FECFrame=Normal  CodeRateSource=Property  CodeRateNormal=1/4  CodeRateShort=1/4  Parallelism=45  Algorithm=Min-sum  SourceScalingFactor=Property  ScalingFactor=0.75  Termination=Max  SpecifyInputs=Property  NumIterations=8  MaxNumIterations=8  ParityCheckStatus=off  SimulateUsing=Code generation
  Logical Operator2 : Logic  AllPortsSameDT=off  OutDataTypeStr=boolean
  Logical Operator3 : Logic  Operator=NOT  AllPortsSameDT=off  OutDataTypeStr=boolean
  Logical Operator4 : Logic  AllPortsSameDT=off  OutDataTypeStr=boolean
  Logical Operator5 : Logic  Operator=NOT  AllPortsSameDT=off  OutDataTypeStr=boolean
  Sample Control Bus Creator : whdlutilities/Sample Control Bus Creator
  bitsOut : Outport
  ctrl : Outport  Port=2
  LDPCFrameIgnored : Outport  Port=3
  BCHFrameIgnored : Outport  Port=4
  wires:
  DVB-S2 LDPC Decoder/2 -> DVB-S2 BCH Decoder/2, Bus Selector/1
  Sample Control Bus Creator/1 -> DVB-S2 LDPC Decoder/2
  startIn/1 -> Sample Control Bus Creator/1, Logical Operator2/1
  DVB-S2 BCH Decoder/3 -> Logical Operator5/1
  DVB-S2 LDPC Decoder/3 -> Logical Operator3/1
  Bus Selector/1 -> Logical Operator4/1  "<start>"
  Logical Operator5/1 -> Logical Operator4/2
  Logical Operator3/1 -> Logical Operator2/2
  DVB-S2 LDPC Decoder/1 -> DVB-S2 BCH Decoder/1
  Logical Operator2/1 -> LDPCFrameIgnored/1
  dataIn/1 -> DVB-S2 LDPC Decoder/1
  endIn/1 -> Sample Control Bus Creator/2
  DVB-S2 BCH Decoder/1 -> bitsOut/1
  validIn/1 -> Sample Control Bus Creator/3
  Logical Operator4/1 -> BCHFrameIgnored/1
  FECFrame/1 -> DVB-S2 LDPC Decoder/3
  codIdx/1 -> DVB-S2 BCH Decoder/3, DVB-S2 LDPC Decoder/4
  DVB-S2 BCH Decoder/2 -> ctrl/1

== system soc_dvbs2_fpga/DVBS2/DVBS2 TxRx/DVB-S2 HDL Receiver/Demod Deinterleave and FECDecode/Symbol Demodulaor ==
  dataIn : Inport
  validIn : Inport  Port=2
  nVarIn : Inport  Port=3
  paramCapture : Inport  Port=4
  modIdx : Inport  Port=5
  codIdx : Inport  Port=6
  FECFrame : Inport  Port=7
  DVBS2 Symbol Demodulator : whdlmod/DVB-S2 Symbol Demodulator  ModulationSourceParams=Input port  ModulationScheme=QPSK  CodeRateAPSK=3/4  DecisionType=Approximate log-likelihood ratio  OutputType=Scalar  UnitAveragePower=off  EnbNoiseVar=off  SimulateUsing=Code generation
  Data Type Conversion : DataTypeConversion  OutDataTypeStr=fixdt(0,3,0)  SaturateOnIntegerOverflow=off  RndMeth=Floor
  Delay : Delay  DelayLength=1
  Delay{1..4} (4 alike) : Delay  DelayLength=15
  Logical Operator : Logic  AllPortsSameDT=off  OutDataTypeStr=boolean
  Logical Operator1 : Logic  Operator=NOT  AllPortsSameDT=off  OutDataTypeStr=boolean
  Terminator : Terminator
  softBitsOut : Outport
  validOut : Outport  Port=2
  paramCaptureOut : Outport  Port=3
  modIdxOut : Outport  Port=4
  codIdxOut : Outport  Port=5
  fecframeOut : Outport  Port=6
  symbolIgnored : Outport  Port=7
  wires:
  codIdx/1 -> Delay2/1, DVBS2 Symbol Demodulator/4
  Delay2/1 -> codIdxOut/1
  modIdx/1 -> Data Type Conversion/1, Delay1/1
  dataIn/1 -> DVBS2 Symbol Demodulator/1
  paramCapture/1 -> Delay4/1
  Data Type Conversion/1 -> DVBS2 Symbol Demodulator/3
  Delay4/1 -> paramCaptureOut/1
  Delay1/1 -> modIdxOut/1
  DVBS2 Symbol Demodulator/2 -> validOut/1
  DVBS2 Symbol Demodulator/1 -> softBitsOut/1
  FECFrame/1 -> Delay3/1
  Delay3/1 -> fecframeOut/1
  validIn/1 -> Logical Operator/1, DVBS2 Symbol Demodulator/2
  Logical Operator1/1 -> Logical Operator/2
  Delay/1 -> Logical Operator1/1
  DVBS2 Symbol Demodulator/3 -> Delay/1
  Logical Operator/1 -> symbolIgnored/1
  nVarIn/1 -> Terminator/1

== system soc_dvbs2_fpga/DVBS2/DVBS2 TxRx/DVB-S2 HDL Receiver/No HDL/Constellation1 ==
  symbSyncOut : Inport
  Enable : EnablePort
  Constellation Plots1 : ConstellationDiagram  WindowPosition=[544.000000,269.000000,286.000000,338.000000,]  ScopeFrameLocation=window  SymbolsToDisplaySource=Property  SymbolsToDisplay=1000  ReferenceConstellation="[0.70711+0.70711i        -0.70711+0.70711i        -0.70711-0.70711i         0.70711-0.70711i]"  ReferenceMarker={''+'',''+''}  ReferenceColor={[1 0 0],[0.0588235294117647 1 1]}  XLimits=[-1.39,1.39]  YLimits=[-1.39,1.39]  AxesLimits=[-1.39,1.39]  ShowLegend=on  DefaultConfigurationName=comm.scopes.ConstellationDiagramBlockCfg
      settings: OpenAtSimulationStart=off
  Data Type Conversion2 : DataTypeConversion  OutDataTypeStr=double  SaturateOnIntegerOverflow=off  RndMeth=Floor
  wires:
  Data Type Conversion2/1 -> Constellation Plots1/1  "Symbol Synchronized Symbols"
  symbSyncOut/1 -> Data Type Conversion2/1

== system soc_dvbs2_fpga/DVBS2/DVBS2 TxRx/DVB-S2 HDL Receiver/No HDL/Constellation2 ==
  symbDemodIndata : Inport
  Enable : EnablePort
  Constellation Plots2 : ConstellationDiagram  WindowPosition=[833.000000,267.000000,279.000000,338.000000,]  ScopeFrameLocation=window  SymbolsToDisplaySource=Property  SymbolsToDisplay=1000  XLimits=[-1.5,1.5]  YLimits=[-1.5,1.5]  AxesLimits=[-1.5,1.5]  ShowLegend=on  DefaultConfigurationName=comm.scopes.ConstellationDiagramBlockCfg
      settings: OpenAtSimulationStart=off
  Data Type Conversion1 : DataTypeConversion  OutDataTypeStr=double  SaturateOnIntegerOverflow=off  RndMeth=Floor
  wires:
  Data Type Conversion1/1 -> Constellation Plots2/1  "Synchronized Data Symbols"
  symbDemodIndata/1 -> Data Type Conversion1/1

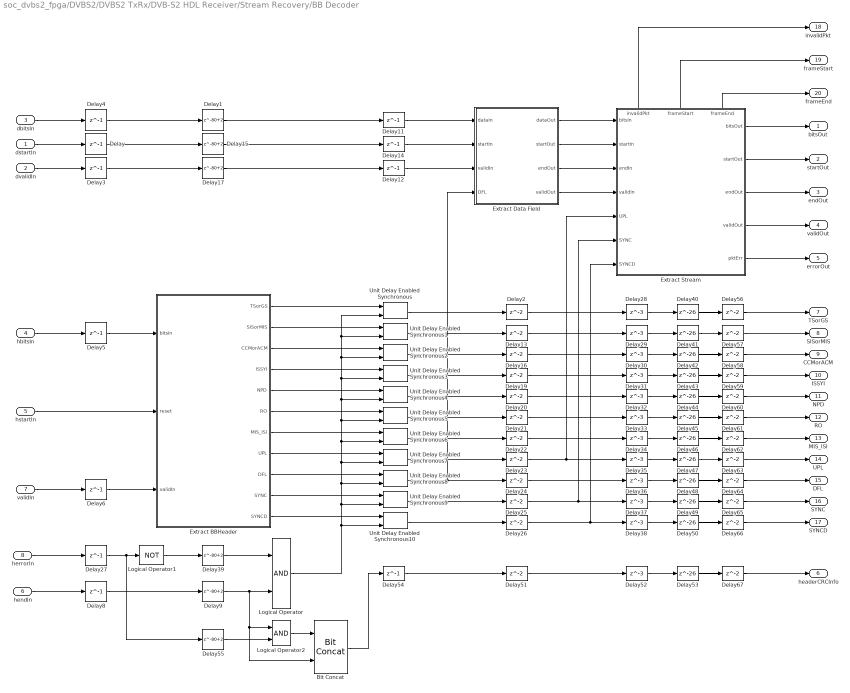
== system soc_dvbs2_fpga/DVBS2/DVBS2 TxRx/DVB-S2 HDL Receiver/Stream Recovery/BB Decoder ==
  dstartIn : Inport
  dvalidIn : Inport  Port=2
  dbitsIn : Inport  Port=3
  hbitsIn : Inport  Port=4
  hstartIn : Inport  Port=5
  hendIn : Inport  Port=6
  validIn : Inport  Port=7
  herrorIn : Inport  Port=8
  Bit Concat : hdlsllib/Logic and Bit Operations/Bit Concat  numInputs=2
  Delay{,3..6,8,11..12,14,27,54} (11 alike) : Delay  DelayLength=1
  Delay{1,9,15,17,39,55} (6 alike) : Delay  DelayLength=80+2
  Delay{2,13,16,19..26,51,56..67} (24 alike) : Delay
  Delay{28..38,52} (12 alike) : Delay  DelayLength=3
  Delay{40..50,53} (12 alike) : Delay  DelayLength=26
  Extract BBHeader : Subsystem
      mask init:
      | subsystems = {'MATYPE2','UPL','DFL','SYNC','SYNCD'};
      | 
      | for ii = 1 : length(subsystems)
      |     Simulink.suppressDiagnostic([gcb '/Extract ' subsystems{ii} '/Add'], 'SimulinkFixedPoint:util:Overflowoccurred');
      |     Simulink.suppressDiagnostic([gcb '/Extract ' subsystems{ii} '/Gain'], 'SimulinkFixedPoint:util:Overflowoccurred');
      | end
  Extract Data Field : Subsystem
  Extract Stream : Subsystem
      settings: PortSchema="{\"entries\":[{\"content\":{\"sides\":[{\"content\":{\"connectorIds\":[\"In1\",\"In2\",\"In3\",\"In4\",\"In5\",\"In6\",\"In7\"]},\"type\":\"ConnectorPlacement.EquallySpacedRectSide\",\"uuid\":\"408fc0bd-98b1-483e-b3dd-853907da4029\"},{\"content\":{\"connectorIds\":[\"Out1\",\"Out2\",\"Out3\",\"Out4\",\"Out5\"],\"side\":\"RIGHT\"},\"type\":\"ConnectorPlacement.EquallySpacedRectSide\",\"uuid\":\"8c197856-6e4f-403e-b137-06ecb7d39191\"},{\"content\":{\"connectorIds\":[\"Out6\",\"Out7\",\"Out8\"],\"side\":\"TOP\"},\"type\":\"ConnectorPlacement.EquallySpacedRectSide\",\"uuid\":\"956083dc-6f9e-45c3-8946-397034fa6e0f\"}]},\"type\":\"ConnectorPlacement.EquallySpacedConnector\",\"uuid\":\"0b4cd761-af75-4bf8-a597-6f9a29b7463a\"}],\"packageUris\":[\"http://schema.mathworks.com/mf0/Connector/R2020b\"],\"version\":\"1.0\"}"
  Logical Operator : Logic  AllPortsSameDT=off  OutDataTypeStr=boolean
  Logical Operator1 : Logic  Operator=NOT  AllPortsSameDT=off  OutDataTypeStr=boolean
  Logical Operator2 : Logic  AllPortsSameDT=off  OutDataTypeStr=boolean
  Unit Delay Enabled Synchronous{,1..10} (11 alike) : hdlsllib/Discrete/Unit Delay Enabled Synchronous  InitialCondition=0.0  SampleTime=-1
  bitsOut : Outport
  startOut : Outport  Port=2
  endOut : Outport  Port=3
  validOut : Outport  Port=4
  errorOut : Outport  Port=5
  headerCRCInfo : Outport  Port=6
  TSorGS : Outport  Port=7
  SISorMIS : Outport  Port=8
  CCMorACM : Outport  Port=9
  ISSYI : Outport  Port=10
  NPD : Outport  Port=11
  RO : Outport  Port=12
  MIS_ISI : Outport  Port=13
  UPL : Outport  Port=14
  DFL : Outport  Port=15
  SYNC : Outport  Port=16
  SYNCD : Outport  Port=17
  invalidPkt : Outport  Port=18
  frameStart : Outport  Port=19
  frameEnd : Outport  Port=20
  wires:
  Extract Stream/5(pktErr) -> errorOut/1
  Extract Stream/4(validOut) -> validOut/1
  Extract Stream/3(endOut) -> endOut/1
  Extract Stream/2(startOut) -> startOut/1
  Extract Stream/1(bitsOut) -> bitsOut/1
  Extract Data Field/4(validOut) -> Extract Stream/4(validIn)
  Extract Data Field/3(endOut) -> Extract Stream/3(endIn)
  Extract Data Field/2(startOut) -> Extract Stream/2(startIn)
  Extract Data Field/1(dataOut) -> Extract Stream/1(bitsIn)
  Delay50/1 -> Delay66/1
  Delay49/1 -> Delay65/1
  Delay48/1 -> Delay64/1
  Delay47/1 -> Delay63/1
  Delay46/1 -> Delay62/1
  Delay45/1 -> Delay61/1
  Delay44/1 -> Delay60/1
  Delay43/1 -> Delay59/1
  Delay42/1 -> Delay58/1
  Delay41/1 -> Delay57/1
  Delay40/1 -> Delay56/1
  Delay38/1 -> Delay50/1
  Delay37/1 -> Delay49/1
  Delay36/1 -> Delay48/1
  Delay35/1 -> Delay47/1
  Delay34/1 -> Delay46/1
  Delay33/1 -> Delay45/1
  Delay32/1 -> Delay44/1
  Delay31/1 -> Delay43/1
  Delay30/1 -> Delay42/1
  Delay29/1 -> Delay41/1
  Delay28/1 -> Delay40/1
  Unit Delay Enabled Synchronous7/1 -> Delay23/1
  Delay26/1 -> Delay38/1, Extract Stream/7(SYNCD)
  Unit Delay Enabled Synchronous10/1 -> Delay26/1
  Delay25/1 -> Extract Stream/6(SYNC), Delay37/1
  Unit Delay Enabled Synchronous9/1 -> Delay25/1
  Delay24/1 -> Delay36/1
  Delay23/1 -> Delay35/1, Extract Stream/5(UPL)
  Delay22/1 -> Delay34/1
  Unit Delay Enabled Synchronous6/1 -> Delay22/1
  Delay21/1 -> Delay33/1
  Unit Delay Enabled Synchronous5/1 -> Delay21/1
  Delay20/1 -> Delay32/1
  Unit Delay Enabled Synchronous4/1 -> Delay20/1
  Delay2/1 -> Delay28/1
  Delay13/1 -> Delay29/1
  Delay16/1 -> Delay30/1
  Unit Delay Enabled Synchronous2/1 -> Delay16/1
  Delay19/1 -> Delay31/1
  Unit Delay Enabled Synchronous3/1 -> Delay19/1
  Unit Delay Enabled Synchronous1/1 -> Delay13/1
  Unit Delay Enabled Synchronous/1 -> Delay2/1
  Delay12/1 -> Extract Data Field/3(validIn)
  Delay14/1 -> Extract Data Field/2(startIn)
  Delay11/1 -> Extract Data Field/1(dataIn)
  Unit Delay Enabled Synchronous8/1 -> Extract Data Field/4(DFL), Delay24/1
  Logical Operator/1 -> Unit Delay Enabled Synchronous10/2, Unit Delay Enabled Synchronous9/2, Unit Delay Enabled Synchronous8/2, Unit Delay Enabled Synchronous7/2, Unit Delay Enabled Synchronous6/2, Unit Delay Enabled Synchronous5/2, Unit Delay Enabled Synchronous4/2, Unit Delay Enabled Synchronous3/2, Unit Delay Enabled Synchronous2/2, Unit Delay Enabled Synchronous1/2, Unit Delay Enabled Synchronous/2
  Extract BBHeader/11(SYNCD) -> Unit Delay Enabled Synchronous10/1
  Extract BBHeader/10(SYNC) -> Unit Delay Enabled Synchronous9/1
  Extract BBHeader/9(DFL) -> Unit Delay Enabled Synchronous8/1
  Extract BBHeader/8(UPL) -> Unit Delay Enabled Synchronous7/1
  Extract BBHeader/7(MIS_ISI) -> Unit Delay Enabled Synchronous6/1
  Extract BBHeader/6(RO) -> Unit Delay Enabled Synchronous5/1
  Extract BBHeader/5(NPD) -> Unit Delay Enabled Synchronous4/1
  Extract BBHeader/4(ISSYI) -> Unit Delay Enabled Synchronous3/1
  Extract BBHeader/3(CCMorACM) -> Unit Delay Enabled Synchronous2/1
  Delay8/1 -> Delay9/1
  hendIn/1 -> Delay8/1
  Delay6/1 -> Extract BBHeader/3(validIn)
  Delay5/1 -> Extract BBHeader/1(bitsIn)
  Delay4/1 -> Delay1/1
  Delay3/1 -> Delay17/1
  Delay/1 -> Delay15/1
  Delay1/1 -> Delay11/1
  dbitsIn/1 -> Delay4/1
  Delay15/1 -> Delay14/1
  Delay17/1 -> Delay12/1
  Extract BBHeader/1(TSorGS) -> Unit Delay Enabled Synchronous/1
  validIn/1 -> Delay6/1
  Extract BBHeader/2(SISorMIS) -> Unit Delay Enabled Synchronous1/1
  dvalidIn/1 -> Delay3/1
  hbitsIn/1 -> Delay5/1
  dstartIn/1 -> Delay/1
  herrorIn/1 -> Delay27/1
  hstartIn/1 -> Extract BBHeader/2(reset)
  Extract Stream/6(invalidPkt) -> invalidPkt/1
  Logical Operator1/1 -> Delay39/1
  Delay27/1 -> Delay55/1, Logical Operator1/1
  Delay39/1 -> Logical Operator/1
  Delay54/1 -> Delay51/1
  Delay51/1 -> Delay52/1
  Delay52/1 -> Delay53/1
  Delay53/1 -> Delay67/1
  Delay55/1 -> Logical Operator2/2
  Delay9/1 -> Logical Operator2/1, Bit Concat/2, Logical Operator/2
  Logical Operator2/1 -> Bit Concat/1
  Bit Concat/1 -> Delay54/1
  Delay56/1 -> TSorGS/1
  Delay57/1 -> SISorMIS/1
  Delay58/1 -> CCMorACM/1
  Delay59/1 -> ISSYI/1
  Delay60/1 -> NPD/1
  Delay61/1 -> RO/1
  Delay62/1 -> MIS_ISI/1
  Delay63/1 -> UPL/1
  Delay64/1 -> DFL/1
  Delay65/1 -> SYNC/1
  Delay66/1 -> SYNCD/1
  Delay67/1 -> headerCRCInfo/1
  Extract Stream/7(frameStart) -> frameStart/1
  Extract Stream/8(frameEnd) -> frameEnd/1

== system soc_dvbs2_fpga/DVBS2/DVBS2 TxRx/DVB-S2 HDL Receiver/Stream Recovery/BB Demultiplexer ==
  bitsIn : Inport
  startIn : Inport  Port=2
  validIn : Inport  Port=3
  Compare To Constant : simulink/Logic and Bit Operations/Compare To Constant  relop=<=  const=80 - 1  OutDataTypeStr=boolean
  Compare To Constant1 : simulink/Logic and Bit Operations/Compare To Constant  relop===  const=80 - 1  OutDataTypeStr=boolean
  Compare To Constant2 : simulink/Logic and Bit Operations/Compare To Constant  relop===  const=80  OutDataTypeStr=boolean
  Delay1 : Delay  DelayLength=1
  Delay2 : Delay  DelayLength=1
  Delay3 : Delay  DelayLength=1
  HDL Counter : hdlsllib/Sources/HDL Counter  CountType=Free running  CountInit=0  CountStep=1  CountMax=25  CountFromType=Initial value  CountFrom=0  CountResetPort=on  CountLoadPort=off  CountEnbPort=on  CountDirPort=off  CountHitOutputPort=off  CountDataType=Unsigned  CountWordLen=nextpow2(58192)  CountFracLen=0  CountSampTime=-1
  Logical Operator{,1,3..4} (4 alike) : Logic  AllPortsSameDT=off  OutDataTypeStr=boolean
  Logical Operator2 : Logic  Operator=NOT  AllPortsSameDT=off  OutDataTypeStr=boolean
  dstartOut : Outport
  dValidOut : Outport  Port=2
  bitsOut : Outport  Port=3
  hstartOut : Outport  Port=4
  hendOut : Outport  Port=5
  hvalidOut : Outport  Port=6
  wires:
  Logical Operator4/1 -> dstartOut/1
  Compare To Constant2/1 -> Logical Operator4/1
  HDL Counter/1 -> Compare To Constant/1, Compare To Constant1/1, Compare To Constant2/1
  Delay3/1 -> HDL Counter/2, Logical Operator/2, Logical Operator3/2, Logical Operator1/2, Logical Operator4/2
  Logical Operator2/1 -> Logical Operator3/1
  Logical Operator3/1 -> dValidOut/1
  Compare To Constant1/1 -> Logical Operator1/1
  Logical Operator1/1 -> hendOut/1
  validIn/1 -> Delay3/1
  bitsIn/1 -> Delay2/1
  Logical Operator/1 -> hvalidOut/1
  Delay2/1 -> bitsOut/1
  startIn/1 -> HDL Counter/1, Delay1/1
  Compare To Constant/1 -> Logical Operator/1, Logical Operator2/1
  Delay1/1 -> hstartOut/1

== system soc_dvbs2_fpga/DVBS2/DVBS2 TxRx/DVB-S2 HDL Receiver/Stream Recovery/BB Descrambler ==
  bitsIn : Inport
  startIn : Inport  Port=2
  validIn : Inport  Port=3
  Data Type Conversion : DataTypeConversion  OutDataTypeStr=boolean  SaturateOnIntegerOverflow=off  RndMeth=Floor
  Logical Operator : Logic  Operator=XOR  AllPortsSameDT=off  OutDataTypeStr=boolean
  Subsystem : Subsystem
  bitsOut : Outport
  startOut : Outport  Port=2
  validOut : Outport  Port=3
  wires:
  bitsIn/1 -> Logical Operator/2
  validIn/1 -> Subsystem/Enable, validOut/1
  Subsystem/1(Out1) -> Data Type Conversion/1
  startIn/1 -> Subsystem/1(In1), startOut/1
  Logical Operator/1 -> bitsOut/1
  Data Type Conversion/1 -> Logical Operator/1
